simulink model "ImageBasedMdlv1"  (R2018a)
settings: Solver=VariableStepAuto  StartTime=0.0  StopTime=10.0  RelTol=1e-3
settings Model: Creator=admin  LastModifiedBy=admin

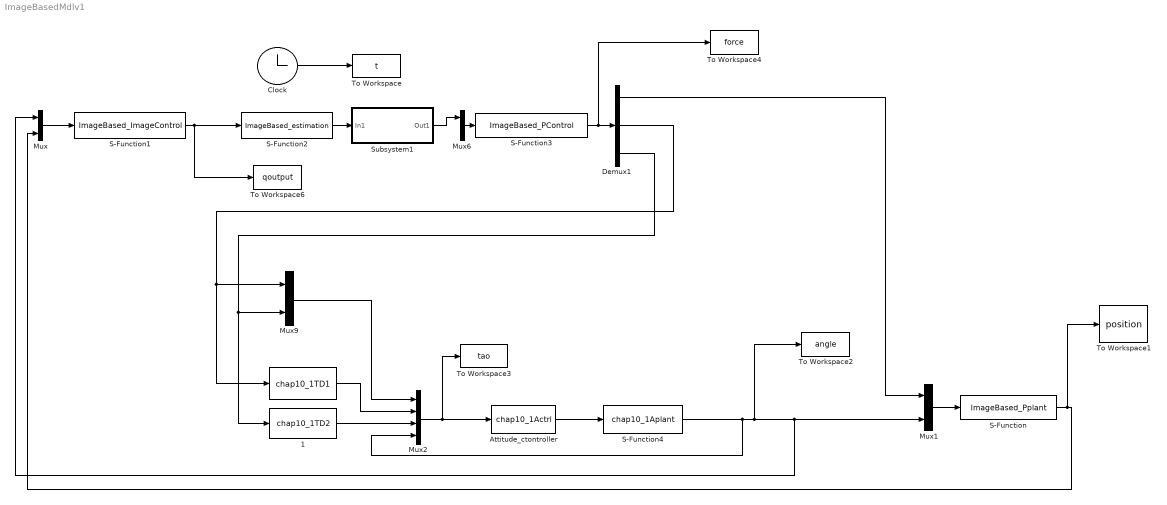
== system ImageBasedMdlv1 ==
  " " : S-Function  FunctionName=chap10_1TD1  SFunctionDeploymentMode=off  EnableBusSupport=off
  " 1" : S-Function  FunctionName=chap10_1TD2  SFunctionDeploymentMode=off  EnableBusSupport=off
  Attitude_ctontroller : S-Function  FunctionName=chap10_1Actrl  SFunctionDeploymentMode=off  EnableBusSupport=off
  Clock : Clock
  Demux1 : Demux  Outputs=3
  Mux{,1,6,9} (4 alike) : Mux  Inputs=2
  Mux2 : Mux
  S-Function : S-Function  FunctionName=ImageBased_Pplant  SFunctionDeploymentMode=off  EnableBusSupport=off
  S-Function1 : S-Function  FunctionName=ImageBased_ImageControl  SFunctionDeploymentMode=off  EnableBusSupport=off
  S-Function2 : S-Function  FunctionName=ImageBased_estimation  SFunctionDeploymentMode=off  EnableBusSupport=off
  S-Function3 : S-Function  FunctionName=ImageBased_PControl  SFunctionDeploymentMode=off  EnableBusSupport=off
  S-Function4 : S-Function  FunctionName=chap10_1Aplant  SFunctionDeploymentMode=off  EnableBusSupport=off
  Subsystem1 : Subsystem
  To Workspace : ToWorkspace  VariableName=t  SampleTime=-1
  To Workspace1 : ToWorkspace  VariableName=position  SampleTime=-1
  To Workspace2 : ToWorkspace  VariableName=angle  SampleTime=-1
  To Workspace3 : ToWorkspace  VariableName=tao  SampleTime=-1
  To Workspace4 : ToWorkspace  VariableName=force  SampleTime=-1
  To Workspace6 : ToWorkspace  VariableName=qoutput  SampleTime=-1
  wires:
  S-Function3/1 -> To Workspace4/1, Demux1/1
  Demux1/1 -> Mux1/1
  S-Function2/1 -> Subsystem1/1(In1)
  S-Function1/1 -> To Workspace6/1, S-Function2/1
  S-Function/1 -> Mux/2, To Workspace1/1
  Mux/1 -> S-Function1/1
  Mux1/1 -> S-Function/1
  Clock/1 -> To Workspace/1
  Subsystem1/1(Out1) -> Mux6/1
  Mux6/1 -> S-Function3/1
  Attitude_ctontroller/1 -> S-Function4/1
  " 1"/1 -> Mux2/3
  Mux9/1 -> Mux2/1
  S-Function4/1 -> Mux2/4, To Workspace2/1, Mux/1, Mux1/2
  " "/1 -> Mux2/2
  Mux2/1 -> To Workspace3/1, Attitude_ctontroller/1
  Demux1/2 -> " "/1, Mux9/1
  Demux1/3 -> " 1"/1, Mux9/2

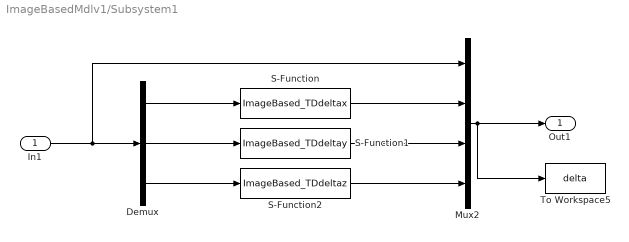
== system ImageBasedMdlv1/Subsystem1 ==
  In1 : Inport
  Demux : Demux  Outputs=3
  Mux2 : Mux
  S-Function : S-Function  FunctionName=ImageBased_TDdeltax  SFunctionDeploymentMode=off  EnableBusSupport=off
  S-Function1 : S-Function  FunctionName=ImageBased_TDdeltay  SFunctionDeploymentMode=off  EnableBusSupport=off
  S-Function2 : S-Function  FunctionName=ImageBased_TDdeltaz  SFunctionDeploymentMode=off  EnableBusSupport=off
  To Workspace5 : ToWorkspace  VariableName=delta  SampleTime=-1
  Out1 : Outport
  wires:
  Demux/3 -> S-Function2/1
  S-Function1/1 -> Mux2/3
  Mux2/1 -> To Workspace5/1, Out1/1
  Demux/1 -> S-Function/1
  Demux/2 -> S-Function1/1
  S-Function/1 -> Mux2/2
  In1/1 -> Mux2/1, Demux/1
  S-Function2/1 -> Mux2/4
